simulink model "two_virtual_wheel_subsystems"  (R2020a)
settings: Solver=VariableStepAuto  StartTime=0.0  StopTime=10.0  RelTol=1e-3
values from neighbouring files (symbols this model uses):
  b1 = T1*k1    (= 0.15)    [two_virtual_wheel_params.m]
  b2 = T2*k2    (= 0.0075)    [two_virtual_wheel_params.m]
  Jw1 = .5*1.5/4    (= 0.1875)    [two_virtual_wheel_params.m]
  Jw2 = 0.0721    [two_virtual_wheel_params.m]
  k1 = .5*15    (= 7.5)    [two_virtual_wheel_params.m]
  k2 = 3.75    [two_virtual_wheel_params.m]
  step_time = 1    [two_virtual_wheel_params.m]
  Theta_z_0 = 45    [two_virtual_wheel_params.m]
undefined symbols (not defined in the file or in its folder): DiscIntNeverNeededParam
libraries: simulink x2
settings Model: Creator=ecs  LastModifiedBy=ecs

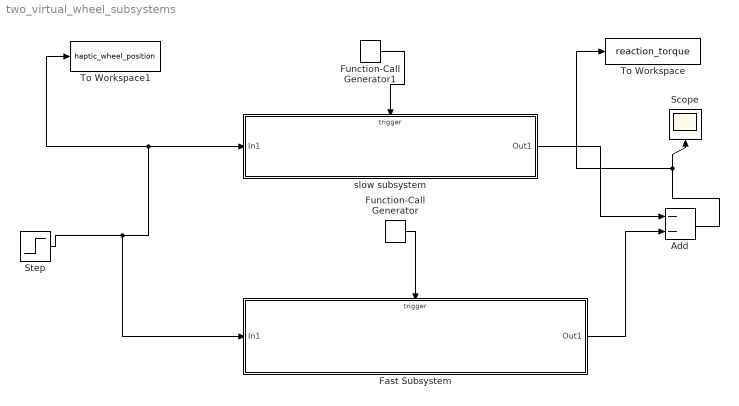
== system two_virtual_wheel_subsystems ==
  Add : Sum  Inputs=--
  Fast Subsystem : Subsystem
  Function-Call Generator : simulink/Ports & Subsystems/Function-Call Generator  sample_time=0.002  numberOfIterations=1
  Function-Call Generator1 : simulink/Ports & Subsystems/Function-Call Generator  sample_time=0.02  numberOfIterations=1
  Scope : Scope
  Step : Step  Time=step_time  After=Theta_z_0  SampleTime=0
  To Workspace : ToWorkspace  VariableName=reaction_torque  SaveFormat=Timeseries  SampleTime=-1
  To Workspace1 : ToWorkspace  VariableName=haptic_wheel_position  SaveFormat=Timeseries  SampleTime=-1
  slow subsystem : Subsystem
  wires:
  Function-Call Generator/1 -> Fast Subsystem/Trigger
  Function-Call Generator1/1 -> slow subsystem/Trigger
  Fast Subsystem/1(Out1) -> Add/2
  slow subsystem/1(Out1) -> Add/1
  Add/1 -> To Workspace/1, Scope/1
  Step/1 -> Fast Subsystem/1(In1), slow subsystem/1(In1), To Workspace1/1

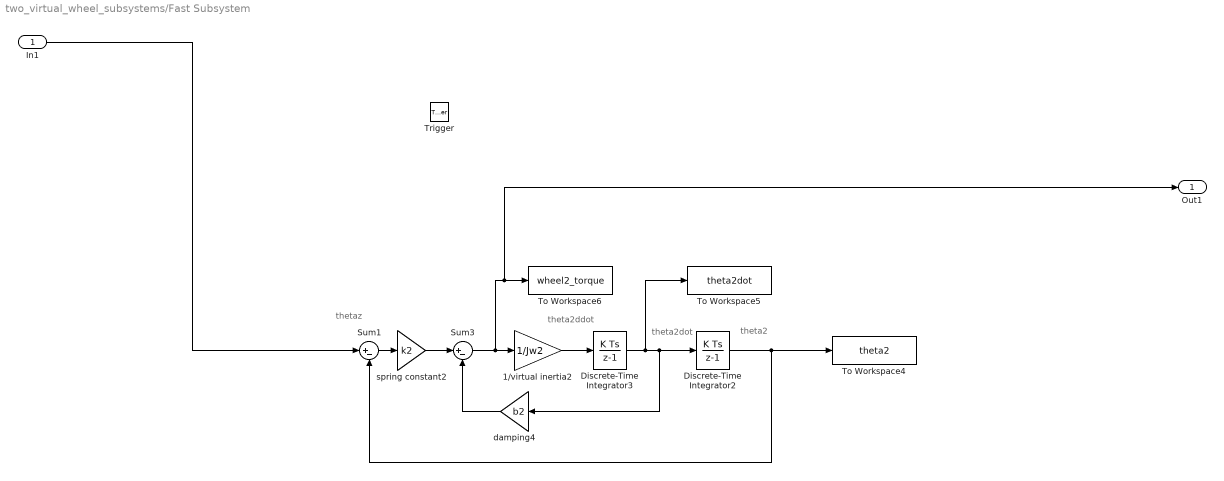
== system two_virtual_wheel_subsystems/Fast Subsystem ==
  note: theta2ddot
  note: thetaz
  note: theta2dot
  note: theta2
  In1 : Inport
  Trigger : TriggerPort  TriggerType=function-call  VariantControl=Variant  PortDimensions=1
  1/virtual inertia2 : Gain  Gain=1/Jw2  SaturateOnIntegerOverflow=on  OutDataTypeStr=Inherit: Same as input  ParamDataTypeStr=Inherit: Same as input
  Discrete-Time Integrator2 : DiscreteIntegrator  SampleTime=-1  ICPrevOutput=DiscIntNeverNeededParam  ICPrevScaledInput=DiscIntNeverNeededParam
  Discrete-Time Integrator3 : DiscreteIntegrator  SampleTime=-1  ICPrevOutput=DiscIntNeverNeededParam  ICPrevScaledInput=DiscIntNeverNeededParam
  Sum1 : Sum  Inputs=|+-  InputSameDT=on  SaturateOnIntegerOverflow=on  OutDataTypeStr=Inherit: Same as first input
  Sum3 : Sum  Inputs=|+-  InputSameDT=on  SaturateOnIntegerOverflow=on  OutDataTypeStr=Inherit: Same as first input
  To Workspace4 : ToWorkspace  VariableName=theta2  SaveFormat=Timeseries  SampleTime=-1
  To Workspace5 : ToWorkspace  VariableName=theta2dot  SaveFormat=Timeseries  SampleTime=-1
  To Workspace6 : ToWorkspace  VariableName=wheel2_torque  SaveFormat=Timeseries  SampleTime=-1
  damping4 : Gain  Gain=b2  SaturateOnIntegerOverflow=on  OutDataTypeStr=Inherit: Same as input  ParamDataTypeStr=Inherit: Same as input
  spring constant2 : Gain  Gain=k2  SaturateOnIntegerOverflow=on  OutDataTypeStr=Inherit: Same as input  ParamDataTypeStr=Inherit: Same as input
  Out1 : Outport
  wires:
  Sum1/1 -> spring constant2/1
  Discrete-Time Integrator3/1 -> To Workspace5/1, Discrete-Time Integrator2/1, damping4/1
  spring constant2/1 -> Sum3/1
  In1/1 -> Sum1/1
  damping4/1 -> Sum3/2
  Discrete-Time Integrator2/1 -> To Workspace4/1, Sum1/2
  Sum3/1 -> 1/virtual inertia2/1, Out1/1, To Workspace6/1
  1/virtual inertia2/1 -> Discrete-Time Integrator3/1

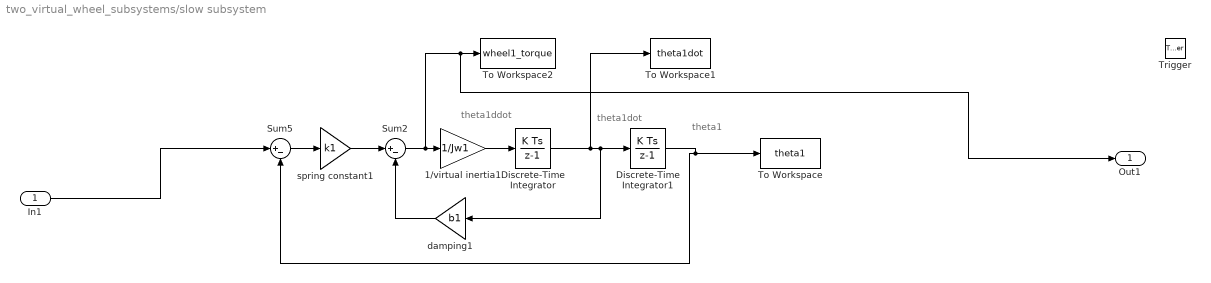
== system two_virtual_wheel_subsystems/slow subsystem ==
  note: theta1ddot
  note: theta1dot
  note: theta1
  In1 : Inport
  Trigger : TriggerPort  TriggerType=function-call  VariantControl=Variant  PortDimensions=1
  1/virtual inertia1 : Gain  Gain=1/Jw1  SaturateOnIntegerOverflow=on  OutDataTypeStr=Inherit: Same as input  ParamDataTypeStr=Inherit: Same as input
  Discrete-Time Integrator : DiscreteIntegrator  SampleTime=-1  ICPrevOutput=DiscIntNeverNeededParam  ICPrevScaledInput=DiscIntNeverNeededParam
  Discrete-Time Integrator1 : DiscreteIntegrator  SampleTime=-1  ICPrevOutput=DiscIntNeverNeededParam  ICPrevScaledInput=DiscIntNeverNeededParam
  Sum2 : Sum  Inputs=|+-  InputSameDT=on  SaturateOnIntegerOverflow=on  OutDataTypeStr=Inherit: Same as first input
  Sum5 : Sum  Inputs=|+-  InputSameDT=on  SaturateOnIntegerOverflow=on  OutDataTypeStr=Inherit: Same as first input
  To Workspace : ToWorkspace  VariableName=theta1  SaveFormat=Timeseries  SampleTime=-1
  To Workspace1 : ToWorkspace  VariableName=theta1dot  SaveFormat=Timeseries  SampleTime=-1
  To Workspace2 : ToWorkspace  VariableName=wheel1_torque  SaveFormat=Timeseries  SampleTime=-1
  damping1 : Gain  Gain=b1  SaturateOnIntegerOverflow=on  OutDataTypeStr=Inherit: Same as input  ParamDataTypeStr=Inherit: Same as input
  spring constant1 : Gain  Gain=k1  SaturateOnIntegerOverflow=on  OutDataTypeStr=Inherit: Same as input  ParamDataTypeStr=Inherit: Same as input
  Out1 : Outport
  wires:
  In1/1 -> Sum5/1
  Sum2/1 -> 1/virtual inertia1/1, Out1/1, To Workspace2/1
  damping1/1 -> Sum2/2
  Sum5/1 -> spring constant1/1
  Discrete-Time Integrator/1 -> Discrete-Time Integrator1/1, damping1/1, To Workspace1/1
  Discrete-Time Integrator1/1 -> Sum5/2, To Workspace/1
  spring constant1/1 -> Sum2/1
  1/virtual inertia1/1 -> Discrete-Time Integrator/1
